simulink subsystem "FPGA"  (R2019b)
settings: Solver=VariableStepAuto  StartTime=0.0  StopTime=10.0  RelTol=1e-3
values from neighbouring files (symbols this model uses):
  ADC_Input_Offset = -0.1139    [RunMe.m]
  ADC_Input_Range = 1.2729    [RunMe.m]
  batches = NumSamples/batchSize    [RunMe.m]
  batchSize = 25    [RunMe.m]
  Bit_Range = 4096    [RunMe.m]
  NumSamples = round(2500e6 * SamplePeriod)    [RunMe.m]
  Output_Shift = 2047    [RunMe.m]
settings Model: Creator=ian  LastModifiedBy=ian

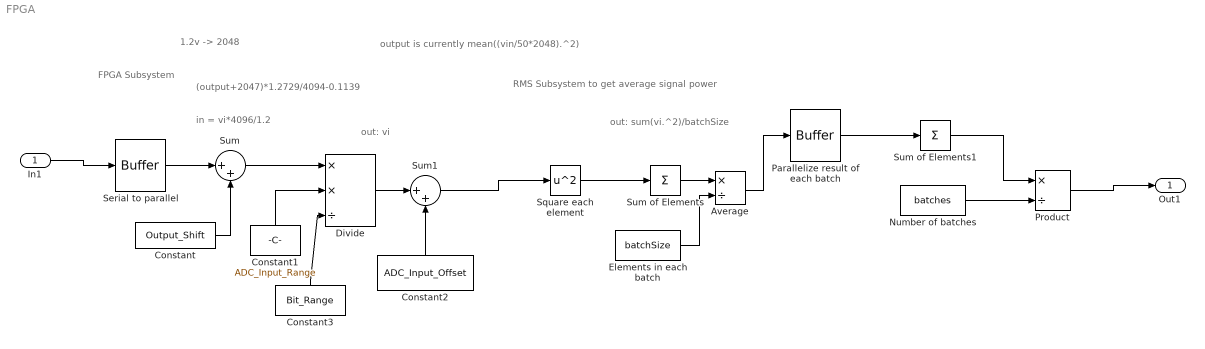
== system FPGA ==
  note: (output+2047)*1.2729/4094-0.1139
  note: out: sum(vi.^2)/batchSize
  note: out: vi
  note: in = vi*4096/1.2
  note: 1.2v -> 2048
  note: output is currently mean((vin/50*2048).^2)
  note: FPGA Subsystem
  note: RMS Subsystem to get average signal power
  In1 : Inport
  Average : Product  Inputs=*/  RndMeth=Zero
  Constant : Constant  Value=Output_Shift  SampleTime=-1
  Constant1 : Constant  Value=ADC_Input_Range  SampleTime=-1
  Constant2 : Constant  Value=ADC_Input_Offset  SampleTime=-1
  Constant3 : Constant  Value=Bit_Range  SampleTime=-1
  Divide : Product  Inputs=**/
  Elements in each batch : Constant  Value=batchSize
  Number of batches : Constant  Value=batches
  Parallelize result of each batch : Buffer  N=batches  OutputFrames=off
  Product : Product  Inputs=*/
  Serial to parallel : Buffer  N=NumSamples/batches  OutputFrames=off
  Square each element : Math  Operator=square  RndMeth=Zero  SaturateOnIntegerOverflow=on
  Sum : Sum  Inputs=|++
  Sum of Elements : Sum  Inputs=+
  Sum of Elements1 : Sum  Inputs=+
  Sum1 : Sum  Inputs=|++
  Out1 : Outport
  wires:
  Average/1 -> Parallelize result of each batch/1
  Elements in each batch/1 -> Average/2
  In1/1 -> Serial to parallel/1
  Sum of Elements/1 -> Average/1
  Square each element/1 -> Sum of Elements/1
  Number of batches/1 -> Product/2
  Parallelize result of each batch/1 -> Sum of Elements1/1
  Product/1 -> Out1/1
  Sum of Elements1/1 -> Product/1
  Constant3/1 -> Divide/3
  Constant1/1 -> Divide/2
  Constant/1 -> Sum/2
  Serial to parallel/1 -> Sum/1
  Sum/1 -> Divide/1
  Divide/1 -> Sum1/1
  Sum1/1 -> Square each element/1
  Constant2/1 -> Sum1/2
